simulink model "SHTL4_TestLevel_4_MODEL"  (R2017b)
settings: Solver=VariableStepAuto  StartTime=0.0  StopTime=80000000  RelTol=1e-3
libraries: instrumentlib x2, svdutilitieslib x1
settings Model: Creator=Bruger  LastModifiedBy=koch

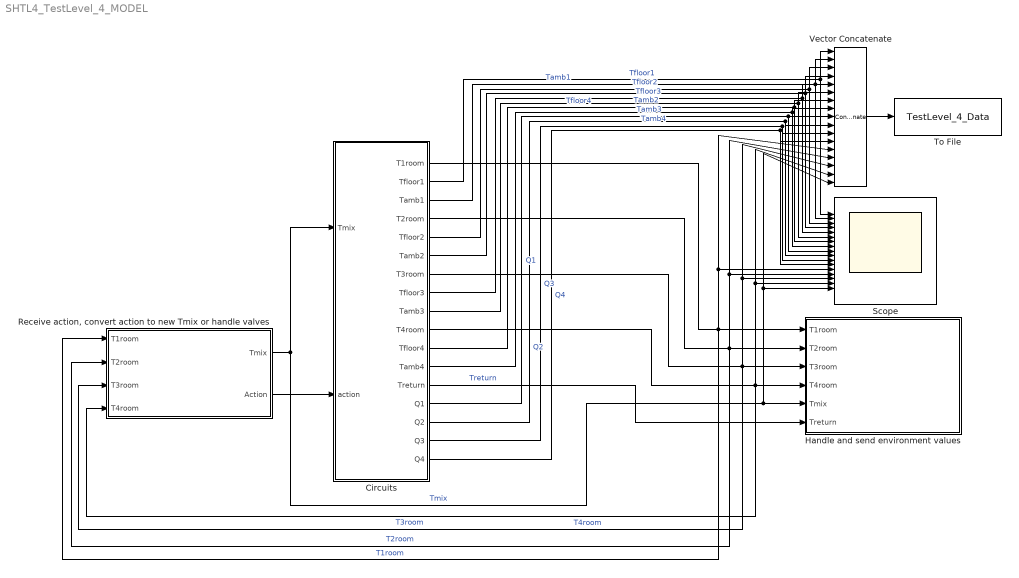
== system SHTL4_TestLevel_4_MODEL ==
  Circuits : Subsystem
  Handle and send environment values : Subsystem
  "Receive action, convert action to new Tmix or handle valves" : Subsystem
  Scope : Scope  NumInputPorts=17
  To File : ToFile  Filename=TestLevel_4_Data  SaveFormat=Timeseries
  Vector Concatenate : Concatenate  NumInputs=17
  wires:
  Vector Concatenate/1 -> To File/1
  "Receive action, convert action to new Tmix or handle valves"/1("Tmix ") -> Scope/17, Vector Concatenate/17, Handle and send environment values/5(Tmix), Circuits/1(Tmix)  "Tmix"
  "Receive action, convert action to new Tmix or handle valves"/2(Action) -> Circuits/2(action)
  Circuits/4(T2room) -> "Receive action, convert action to new Tmix or handle valves"/2(T2room), Scope/14, Vector Concatenate/14, Handle and send environment values/2(T2room)  "T2room"
  Circuits/7(T3room) -> "Receive action, convert action to new Tmix or handle valves"/3(T3room), Scope/15, Vector Concatenate/15, Handle and send environment values/3(T3room)  "T3room"
  Circuits/10(T4room) -> "Receive action, convert action to new Tmix or handle valves"/4(T4room), Scope/16, Vector Concatenate/16, Handle and send environment values/4(T4room)  "T4room"
  Circuits/1(T1room) -> "Receive action, convert action to new Tmix or handle valves"/1(T1room), Scope/13, Vector Concatenate/13, Handle and send environment values/1(T1room)  "T1room"
  Circuits/2(Tfloor1) -> Scope/1, Vector Concatenate/1  "Tfloor1"
  Circuits/3(Tamb1) -> Scope/2, Vector Concatenate/2  "Tamb1"
  Circuits/5(Tfloor2) -> Scope/3, Vector Concatenate/3  "Tfloor2"
  Circuits/6(Tamb2) -> Scope/4, Vector Concatenate/4  "Tamb2"
  Circuits/8(Tfloor3) -> Scope/5, Vector Concatenate/5  "Tfloor3"
  Circuits/9(Tamb3) -> Scope/6, Vector Concatenate/6  "Tamb3"
  Circuits/11(Tfloor4) -> Scope/7, Vector Concatenate/7  "Tfloor4"
  Circuits/12(Tamb4) -> Scope/8, Vector Concatenate/8  "Tamb4"
  Circuits/13(Treturn) -> Handle and send environment values/6(Treturn)  "Treturn"
  Circuits/14(Q1) -> Scope/9, Vector Concatenate/9  "Q1"
  Circuits/15(Q2) -> Scope/10, Vector Concatenate/10  "Q2"
  Circuits/16(Q3) -> Scope/11, Vector Concatenate/11  "Q3"
  Circuits/17(Q4) -> Scope/12, Vector Concatenate/12  "Q4"

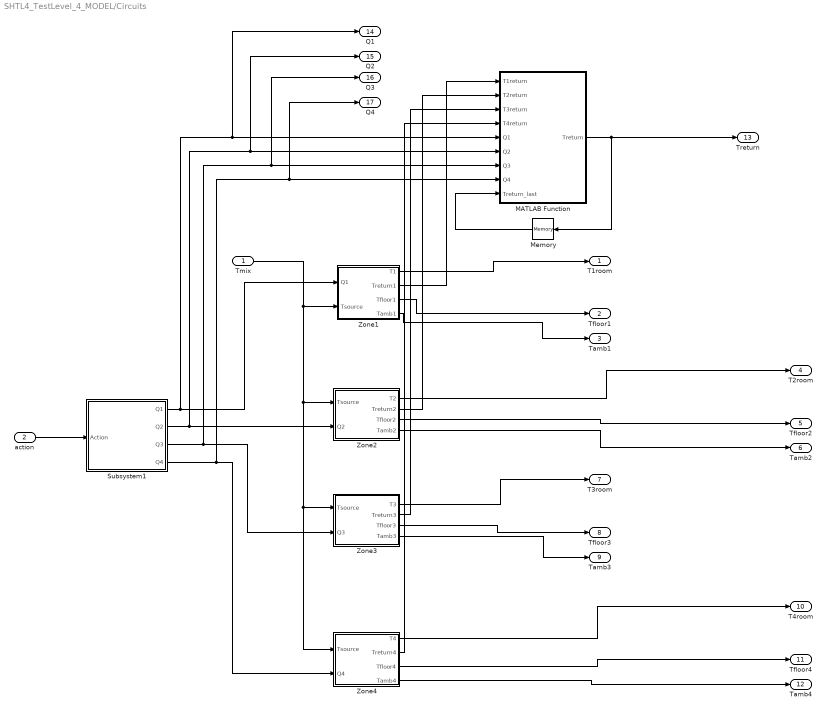
== system SHTL4_TestLevel_4_MODEL/Circuits ==
  Tmix : Inport
  action : Inport  Port=2
  MATLAB Function : MATLAB Function  TreatAsAtomicUnit=on
  Memory : Memory
  Subsystem1 : Subsystem
  Zone1 : Subsystem  Tag=Zone1  Description=Zone1
  Zone2 : Subsystem
  Zone3 : Subsystem
  Zone4 : Subsystem
  T1room : Outport
  Tfloor1 : Outport  Port=2
  Tamb1 : Outport  Port=3
  T2room : Outport  Port=4
  Tfloor2 : Outport  Port=5
  Tamb2 : Outport  Port=6
  T3room : Outport  Port=7
  Tfloor3 : Outport  Port=8
  Tamb3 : Outport  Port=9
  T4room : Outport  Port=10
  Tfloor4 : Outport  Port=11
  Tamb4 : Outport  Port=12
  Treturn : Outport  Port=13
  Q1 : Outport  Port=14
  Q2 : Outport  Port=15
  Q3 : Outport  Port=16
  Q4 : Outport  Port=17
  wires:
  Subsystem1/4("Q4 ") -> Q4/1, MATLAB Function/8(Q4), Zone4/2("Q4 ")
  action/1 -> Subsystem1/1("Action ")
  Tmix/1 -> Zone3/1(Tsource), Zone4/1(Tsource), Zone2/1(Tsource), Zone1/2(Tsource)
  Subsystem1/3(Q3) -> Q3/1, MATLAB Function/7(Q3), Zone3/2("Q3 ")
  Subsystem1/1("Q1 ") -> Q1/1, MATLAB Function/5(Q1), Zone1/1("Q1 ")
  Zone1/1(T1) -> T1room/1
  Zone1/2("Treturn1 ") -> MATLAB Function/1(T1return)
  Subsystem1/2(Q2) -> Q2/1, MATLAB Function/6(Q2), Zone2/2("Q2 ")
  Zone2/2("Treturn2 ") -> MATLAB Function/2(T2return)
  Zone3/2("Treturn3 ") -> MATLAB Function/3(T3return)
  Zone4/2(Treturn4) -> MATLAB Function/4(T4return)
  Zone1/3("Tfloor1 ") -> Tfloor1/1
  Zone1/4("Tamb1 ") -> Tamb1/1
  Zone2/1("T2 ") -> T2room/1
  Zone2/3("Tfloor2 ") -> Tfloor2/1
  Zone2/4("Tamb2 ") -> Tamb2/1
  Zone3/1(T3) -> T3room/1
  Zone3/3(Tfloor3) -> Tfloor3/1
  Zone3/4("Tamb3 ") -> Tamb3/1
  Zone4/1("T4 ") -> T4room/1
  Zone4/3("Tfloor4 ") -> Tfloor4/1
  Zone4/4("Tamb4 ") -> Tamb4/1
  MATLAB Function/1(Treturn) -> Treturn/1, Memory/1
  Memory/1 -> MATLAB Function/9(Treturn_last)

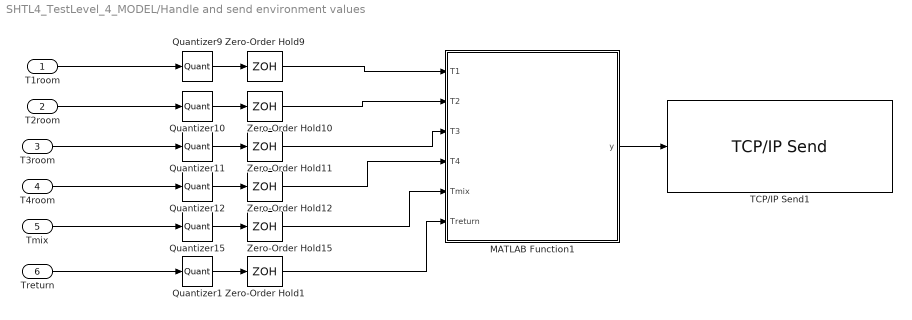
== system SHTL4_TestLevel_4_MODEL/Handle and send environment values ==
  T1room : Inport
  T2room : Inport  Port=2
  T3room : Inport  Port=3
  T4room : Inport  Port=4
  Tmix : Inport  Port=5
  Treturn : Inport  Port=6
  MATLAB Function1 : MATLAB Function  TreatAsAtomicUnit=on
  Quantizer{1,9..12,15} (6 alike) : Quantizer  QuantizationInterval=0.01
  TCP/IP Send1 : instrumentlib/TCP//IP Send  Host=localhost  Port=50001  EnableBlockingMode=on  Timeout=40  ByteOrder=LittleEndian
      settings: SourceProductName=Instrument Control Toolbox
  Zero-Order Hold{1,9..12,15} (6 alike) : ZeroOrderHold  SampleTime=-1
  wires:
  T4room/1 -> Quantizer12/1
  T1room/1 -> Quantizer9/1
  T3room/1 -> Quantizer11/1
  Tmix/1 -> Quantizer15/1
  T2room/1 -> Quantizer10/1
  Zero-Order Hold11/1 -> MATLAB Function1/3(T3)
  Quantizer11/1 -> Zero-Order Hold11/1
  Quantizer12/1 -> Zero-Order Hold12/1
  MATLAB Function1/1(y) -> TCP/IP Send1/1
  Zero-Order Hold10/1 -> MATLAB Function1/2(T2)
  Quantizer15/1 -> Zero-Order Hold15/1
  Zero-Order Hold12/1 -> MATLAB Function1/4(T4)
  Quantizer10/1 -> Zero-Order Hold10/1
  Zero-Order Hold9/1 -> MATLAB Function1/1(T1)
  Quantizer9/1 -> Zero-Order Hold9/1
  Zero-Order Hold15/1 -> MATLAB Function1/5(Tmix)
  Quantizer1/1 -> Zero-Order Hold1/1
  Treturn/1 -> Quantizer1/1
  Zero-Order Hold1/1 -> MATLAB Function1/6(Treturn)

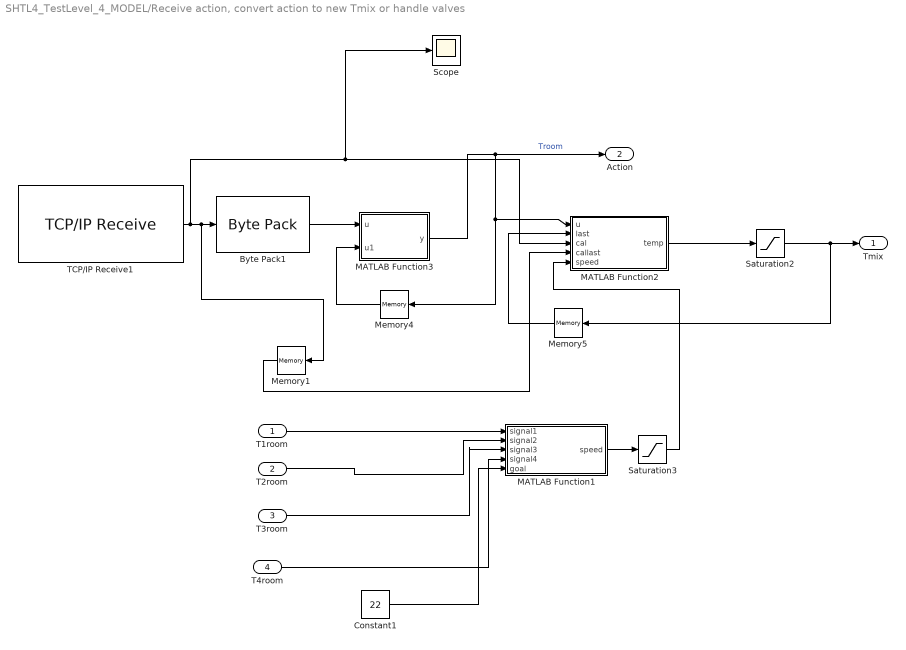
== system SHTL4_TestLevel_4_MODEL/Receive action, convert action to new Tmix or handle valves ==
  T1room : Inport
  T2room : Inport  Port=2
  T3room : Inport  Port=3
  T4room : Inport  Port=4
  Byte Pack1 : svdutilitieslib/Byte Pack  datatypes={'uint8'}  byteAlign=1  blockPlatform=arduinoert
      settings: SourceProductName=Simulink Support Package for Arduino Hardware  SourceProductBaseCode=ARDUINO
  Constant1 : Constant  Value=22
  MATLAB Function1 : MATLAB Function  TreatAsAtomicUnit=on
  MATLAB Function2 : MATLAB Function  TreatAsAtomicUnit=on
  MATLAB Function3 : MATLAB Function  TreatAsAtomicUnit=on
  Memory1 : Memory  InitialCondition=24
  Memory4 : Memory
  Memory5 : Memory  InitialCondition=24
  Saturation2 : Saturate  UpperLimit=45  LowerLimit=15
  Saturation3 : Saturate  UpperLimit=0.8  LowerLimit=0.005
  Scope : Scope
  TCP/IP Receive1 : instrumentlib/TCP//IP Receive  Host=localhost  Port=50000  DataSize=[1 1]  EnableBlockingMode=on  Timeout=40  SampleTime=200  DataType=uint8  ByteOrder=BigEndian
      settings: SourceProductName=Instrument Control Toolbox
  "Tmix " : Outport
  Action : Outport  Port=2
  wires:
  MATLAB Function1/1(speed) -> Saturation3/1
  Saturation3/1 -> MATLAB Function2/5(speed)
  MATLAB Function2/1(temp) -> Saturation2/1
  Byte Pack1/1 -> MATLAB Function3/1(u)
  MATLAB Function3/1(y) -> Action/1, Memory4/1, MATLAB Function2/1(u)  "Troom"
  TCP/IP Receive1/1 -> Scope/1, MATLAB Function2/3(cal), Memory1/1, Byte Pack1/1
  Memory4/1 -> MATLAB Function3/2(u1)
  Constant1/1 -> MATLAB Function1/5(goal)
  Memory5/1 -> MATLAB Function2/2(last)
  T1room/1 -> MATLAB Function1/1(signal1)
  T4room/1 -> MATLAB Function1/4(signal4)
  T3room/1 -> MATLAB Function1/3(signal3)
  T2room/1 -> MATLAB Function1/2(signal2)
  Saturation2/1 -> "Tmix "/1, Memory5/1
  Memory1/1 -> MATLAB Function2/4(callast)

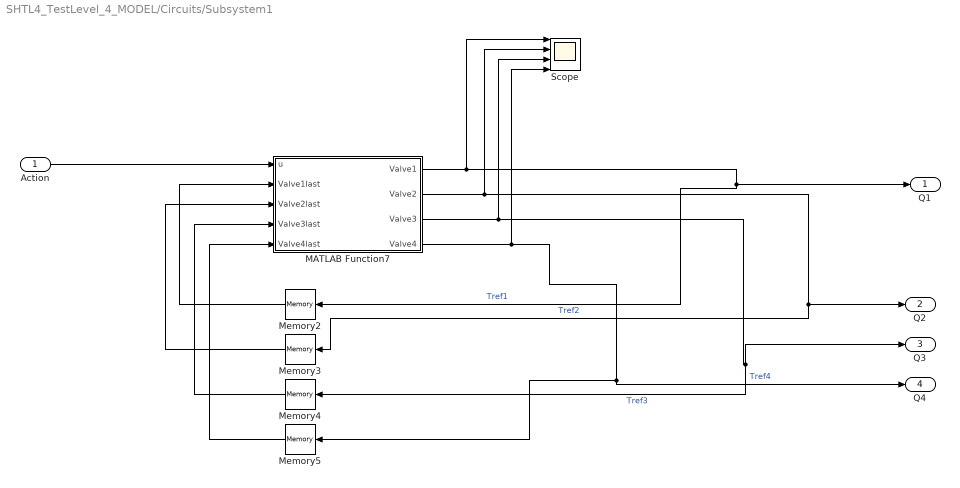
== system SHTL4_TestLevel_4_MODEL/Circuits/Subsystem1 ==
  "Action " : Inport
  MATLAB Function7 : MATLAB Function  TreatAsAtomicUnit=on
  Memory{2..5} (4 alike) : Memory  InitialCondition=0.000027777778
  Scope : Scope  NumInputPorts=4
  "Q1 " : Outport
  Q2 : Outport  Port=2
  Q3 : Outport  Port=3
  "Q4 " : Outport  Port=4
  wires:
  MATLAB Function7/4(Valve4) -> Scope/4, "Q4 "/1, Memory5/1  "Tref4"
  MATLAB Function7/3(Valve3) -> Scope/3, Q3/1, Memory4/1  "Tref3"
  MATLAB Function7/1(Valve1) -> Scope/1, Memory2/1, "Q1 "/1  "Tref1"
  MATLAB Function7/2(Valve2) -> Scope/2, Q2/1, Memory3/1  "Tref2"
  Memory5/1 -> MATLAB Function7/5(Valve4last)
  Memory2/1 -> MATLAB Function7/2(Valve1last)
  Memory4/1 -> MATLAB Function7/4(Valve3last)
  Memory3/1 -> MATLAB Function7/3(Valve2last)
  "Action "/1 -> MATLAB Function7/1(u)

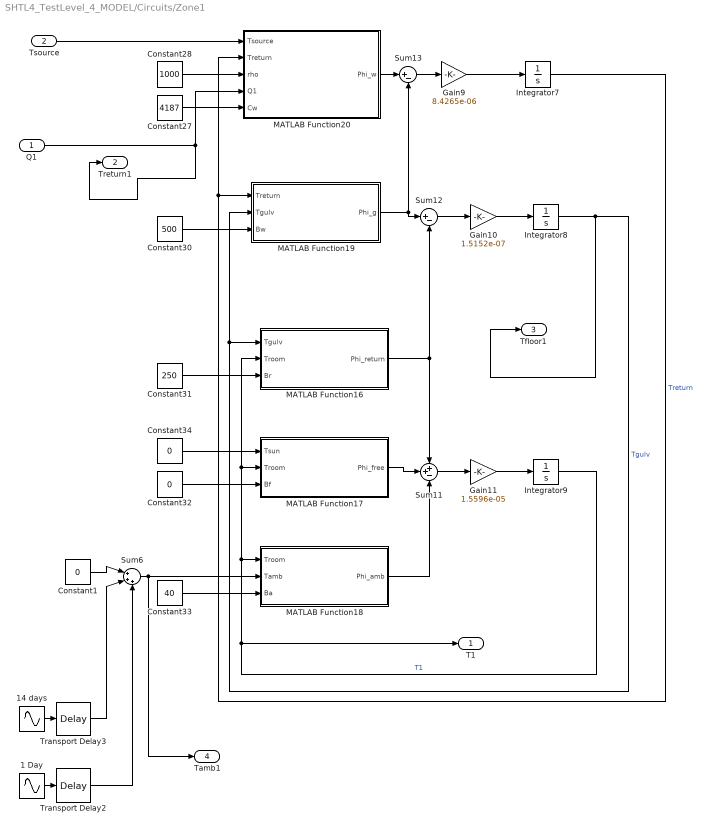
== system SHTL4_TestLevel_4_MODEL/Circuits/Zone1 ==
  "Q1 " : Inport
  Tsource : Inport  Port=2
  1 Day : Sin  Amplitude=4  Frequency=0.00007272205216643  SampleTime=0
  14 days : Sin  Amplitude=2  Frequency=0.00000519443  SampleTime=0
  Constant1 : Constant  Value=0
  Constant27 : Constant  Value=4187
  Constant28 : Constant  Value=1000
  Constant30 : Constant  Value=500
  Constant31 : Constant  Value=250
  Constant32 : Constant  Value=0
  Constant33 : Constant  Value=40
  Constant34 : Constant  Value=0
  Gain10 : Gain  Gain=1.5152e-07
  Gain11 : Gain  Gain=1.5596e-05
  Gain9 : Gain  Gain=8.4265e-06
  Integrator7 : Integrator  InitialCondition=15
  Integrator8 : Integrator  InitialCondition=15
  Integrator9 : Integrator  InitialCondition=15
  MATLAB Function16 : MATLAB Function  TreatAsAtomicUnit=on
  MATLAB Function17 : MATLAB Function  TreatAsAtomicUnit=on
  MATLAB Function18 : MATLAB Function  TreatAsAtomicUnit=on
  MATLAB Function19 : MATLAB Function  TreatAsAtomicUnit=on
  MATLAB Function20 : MATLAB Function  TreatAsAtomicUnit=on
  Sum11 : Sum  Inputs=++-
  Sum12 : Sum  Inputs=|+-
  Sum13 : Sum  Inputs=|+-
  Sum6 : Sum  Inputs=|+++
  Transport Delay2 : TransportDelay  DelayTime=15000000
  Transport Delay3 : TransportDelay  DelayTime=10000000
  T1 : Outport
  "Treturn1 " : Outport  Port=2
  "Tfloor1 " : Outport  Port=3
  "Tamb1 " : Outport  Port=4
  wires:
  Tsource/1 -> MATLAB Function20/1(Tsource)
  MATLAB Function20/1(Phi_w) -> Sum13/1
  Sum12/1 -> Gain10/1
  Constant31/1 -> MATLAB Function16/3(Br)
  Constant32/1 -> MATLAB Function17/3(Bf)
  Integrator7/1 -> MATLAB Function20/2(Treturn), MATLAB Function19/1(Treturn)  "Treturn"
  Gain11/1 -> Integrator9/1
  Constant33/1 -> MATLAB Function18/3(Ba)
  Gain9/1 -> Integrator7/1
  Constant34/1 -> MATLAB Function17/1(Tsun)
  Constant30/1 -> MATLAB Function19/3(Bw)
  Constant27/1 -> MATLAB Function20/5(Cw)
  Integrator9/1 -> T1/1, MATLAB Function16/2(Troom), MATLAB Function17/2(Troom), MATLAB Function18/1(Troom)  "T1"
  MATLAB Function18/1(Phi_amb) -> Sum11/3
  MATLAB Function19/1(Phi_g) -> Sum13/2, Sum12/1
  Sum11/1 -> Gain11/1
  Sum13/1 -> Gain9/1
  Integrator8/1 -> "Tfloor1 "/1, MATLAB Function16/1(Tgulv), MATLAB Function19/2(Tgulv)  "Tgulv"
  MATLAB Function16/1(Phi_return) -> Sum11/1, Sum12/2
  MATLAB Function17/1(Phi_free) -> Sum11/2
  Gain10/1 -> Integrator8/1
  Constant28/1 -> MATLAB Function20/3(rho)
  "Q1 "/1 -> "Treturn1 "/1, MATLAB Function20/4(Q1)
  Transport Delay2/1 -> Sum6/3
  14 days/1 -> Transport Delay3/1
  1 Day/1 -> Transport Delay2/1
  Constant1/1 -> Sum6/1
  Transport Delay3/1 -> Sum6/2
  Sum6/1 -> "Tamb1 "/1, MATLAB Function18/2(Tamb)

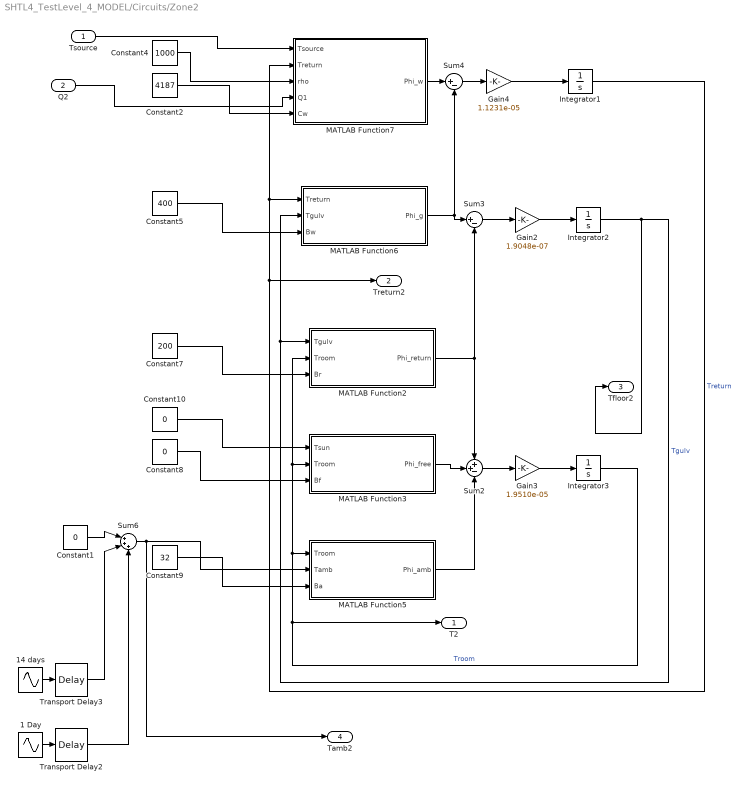
== system SHTL4_TestLevel_4_MODEL/Circuits/Zone2 ==
  Tsource : Inport
  "Q2 " : Inport  Port=2
  1 Day : Sin  Amplitude=4  Frequency=0.00007272205216643  SampleTime=0
  14 days : Sin  Amplitude=2  Frequency=0.00000519443  SampleTime=0
  Constant1 : Constant  Value=0
  Constant10 : Constant  Value=0
  Constant2 : Constant  Value=4187
  Constant4 : Constant  Value=1000
  Constant5 : Constant  Value=400
  Constant7 : Constant  Value=200
  Constant8 : Constant  Value=0
  Constant9 : Constant  Value=32
  Gain2 : Gain  Gain=1.9048e-07
  Gain3 : Gain  Gain=1.9510e-05
  Gain4 : Gain  Gain=1.1231e-05
  Integrator1 : Integrator  InitialCondition=15
  Integrator2 : Integrator  InitialCondition=15
  Integrator3 : Integrator  InitialCondition=15
  MATLAB Function2 : MATLAB Function  TreatAsAtomicUnit=on
  MATLAB Function3 : MATLAB Function  TreatAsAtomicUnit=on
  MATLAB Function5 : MATLAB Function  TreatAsAtomicUnit=on
  MATLAB Function6 : MATLAB Function  TreatAsAtomicUnit=on
  MATLAB Function7 : MATLAB Function  TreatAsAtomicUnit=on
  Sum2 : Sum  Inputs=++-
  Sum3 : Sum  Inputs=|+-
  Sum4 : Sum  Inputs=|+-
  Sum6 : Sum  Inputs=|+++
  Transport Delay2 : TransportDelay  DelayTime=15000000
  Transport Delay3 : TransportDelay  DelayTime=10000000
  "T2 " : Outport
  "Treturn2 " : Outport  Port=2
  "Tfloor2 " : Outport  Port=3
  "Tamb2 " : Outport  Port=4
  wires:
  Gain4/1 -> Integrator1/1
  Gain3/1 -> Integrator3/1
  MATLAB Function5/1(Phi_amb) -> Sum2/3
  Integrator2/1 -> "Tfloor2 "/1, MATLAB Function2/1(Tgulv), MATLAB Function6/2(Tgulv)  "Tgulv"
  Constant2/1 -> MATLAB Function7/5(Cw)
  MATLAB Function7/1(Phi_w) -> Sum4/1
  Sum4/1 -> Gain4/1
  Sum3/1 -> Gain2/1
  Integrator1/1 -> MATLAB Function7/2(Treturn), MATLAB Function6/1(Treturn), "Treturn2 "/1  "Treturn"
  Gain2/1 -> Integrator2/1
  MATLAB Function2/1(Phi_return) -> Sum2/1, Sum3/2
  Constant7/1 -> MATLAB Function2/3(Br)
  MATLAB Function6/1(Phi_g) -> Sum4/2, Sum3/1
  MATLAB Function3/1(Phi_free) -> Sum2/2
  Constant9/1 -> MATLAB Function5/3(Ba)
  Constant4/1 -> MATLAB Function7/3(rho)
  Integrator3/1 -> MATLAB Function2/2(Troom), MATLAB Function3/2(Troom), MATLAB Function5/1(Troom), "T2 "/1  "Troom"
  Sum2/1 -> Gain3/1
  Constant5/1 -> MATLAB Function6/3(Bw)
  "Q2 "/1 -> MATLAB Function7/4(Q1)
  Constant8/1 -> MATLAB Function3/3(Bf)
  Constant10/1 -> MATLAB Function3/1(Tsun)
  Tsource/1 -> MATLAB Function7/1(Tsource)
  Transport Delay2/1 -> Sum6/3
  14 days/1 -> Transport Delay3/1
  1 Day/1 -> Transport Delay2/1
  Constant1/1 -> Sum6/1
  Transport Delay3/1 -> Sum6/2
  Sum6/1 -> "Tamb2 "/1, MATLAB Function5/2(Tamb)

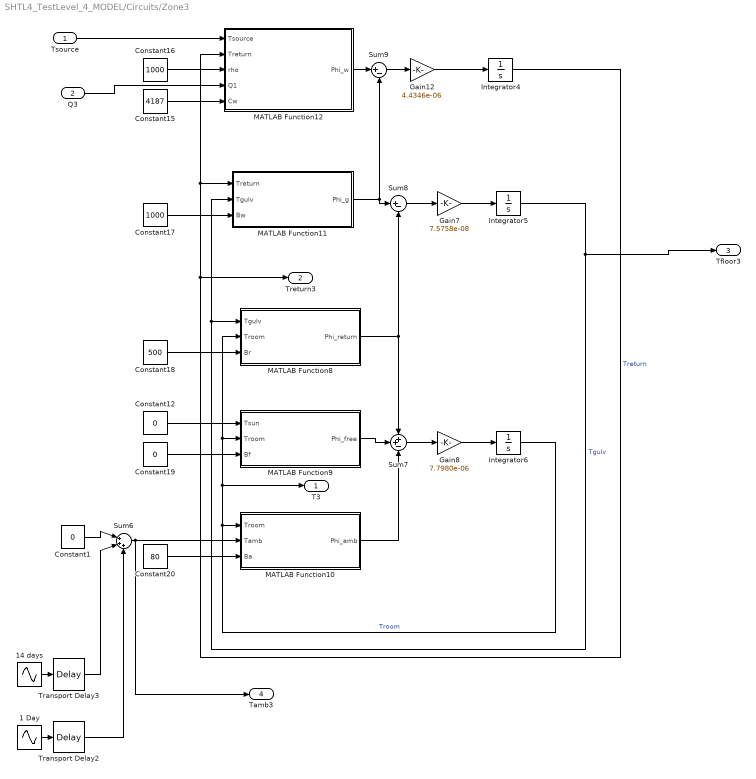
== system SHTL4_TestLevel_4_MODEL/Circuits/Zone3 ==
  Tsource : Inport
  "Q3 " : Inport  Port=2
  1 Day : Sin  Amplitude=4  Frequency=0.00007272205216643  SampleTime=0
  14 days : Sin  Amplitude=2  Frequency=0.00000519443  SampleTime=0
  Constant1 : Constant  Value=0
  Constant12 : Constant  Value=0
  Constant15 : Constant  Value=4187
  Constant16 : Constant  Value=1000
  Constant17 : Constant  Value=1000
  Constant18 : Constant  Value=500
  Constant19 : Constant  Value=0
  Constant20 : Constant  Value=80
  Gain12 : Gain  Gain=4.4346e-06
  Gain7 : Gain  Gain=7.5758e-08
  Gain8 : Gain  Gain=7.7980e-06
  Integrator4 : Integrator  InitialCondition=15
  Integrator5 : Integrator  InitialCondition=15
  Integrator6 : Integrator  InitialCondition=15
  MATLAB Function10 : MATLAB Function  TreatAsAtomicUnit=on
  MATLAB Function11 : MATLAB Function  TreatAsAtomicUnit=on
  MATLAB Function12 : MATLAB Function  TreatAsAtomicUnit=on
  MATLAB Function8 : MATLAB Function  TreatAsAtomicUnit=on
  MATLAB Function9 : MATLAB Function  TreatAsAtomicUnit=on
  Sum6 : Sum  Inputs=|+++
  Sum7 : Sum  Inputs=++-
  Sum8 : Sum  Inputs=|+-
  Sum9 : Sum  Inputs=|+-
  Transport Delay2 : TransportDelay  DelayTime=15000000
  Transport Delay3 : TransportDelay  DelayTime=10000000
  T3 : Outport
  "Treturn3 " : Outport  Port=2
  Tfloor3 : Outport  Port=3
  "Tamb3 " : Outport  Port=4
  wires:
  Constant17/1 -> MATLAB Function11/3(Bw)
  Integrator5/1 -> Tfloor3/1, MATLAB Function8/1(Tgulv), MATLAB Function11/2(Tgulv)  "Tgulv"
  MATLAB Function8/1(Phi_return) -> Sum7/1, Sum8/2
  Sum7/1 -> Gain8/1
  Gain7/1 -> Integrator5/1
  Constant16/1 -> MATLAB Function12/3(rho)
  MATLAB Function11/1(Phi_g) -> Sum9/2, Sum8/1
  Gain8/1 -> Integrator6/1
  Constant20/1 -> MATLAB Function10/3(Ba)
  MATLAB Function12/1(Phi_w) -> Sum9/1
  Integrator4/1 -> MATLAB Function12/2(Treturn), MATLAB Function11/1(Treturn), "Treturn3 "/1  "Treturn"
  Sum9/1 -> Gain12/1
  Constant15/1 -> MATLAB Function12/5(Cw)
  MATLAB Function10/1(Phi_amb) -> Sum7/3
  Constant19/1 -> MATLAB Function9/3(Bf)
  "Q3 "/1 -> MATLAB Function12/4(Q1)
  Sum8/1 -> Gain7/1
  Gain12/1 -> Integrator4/1
  Constant18/1 -> MATLAB Function8/3(Br)
  MATLAB Function9/1(Phi_free) -> Sum7/2
  Constant12/1 -> MATLAB Function9/1(Tsun)
  Integrator6/1 -> MATLAB Function10/1(Troom), MATLAB Function8/2(Troom), MATLAB Function9/2(Troom), T3/1  "Troom"
  Tsource/1 -> MATLAB Function12/1(Tsource)
  Transport Delay2/1 -> Sum6/3
  14 days/1 -> Transport Delay3/1
  1 Day/1 -> Transport Delay2/1
  Constant1/1 -> Sum6/1
  Transport Delay3/1 -> Sum6/2
  Sum6/1 -> "Tamb3 "/1, MATLAB Function10/2(Tamb)

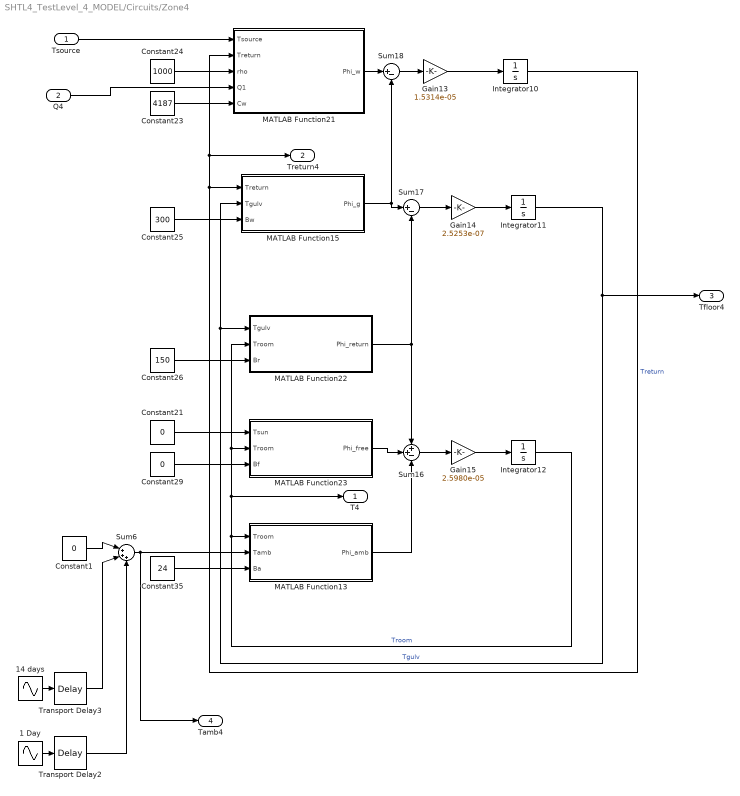
== system SHTL4_TestLevel_4_MODEL/Circuits/Zone4 ==
  Tsource : Inport
  "Q4 " : Inport  Port=2
  1 Day : Sin  Amplitude=4  Frequency=0.00007272205216643  SampleTime=0
  14 days : Sin  Amplitude=2  Frequency=0.00000519443  SampleTime=0
  Constant1 : Constant  Value=0
  Constant21 : Constant  Value=0
  Constant23 : Constant  Value=4187
  Constant24 : Constant  Value=1000
  Constant25 : Constant  Value=300
  Constant26 : Constant  Value=150
  Constant29 : Constant  Value=0
  Constant35 : Constant  Value=24
  Gain13 : Gain  Gain=1.5314e-05
  Gain14 : Gain  Gain=2.5253e-07
  Gain15 : Gain  Gain=2.5980e-05
  Integrator10 : Integrator  InitialCondition=15
  Integrator11 : Integrator  InitialCondition=15
  Integrator12 : Integrator  InitialCondition=15
  MATLAB Function13 : MATLAB Function  TreatAsAtomicUnit=on
  MATLAB Function15 : MATLAB Function  TreatAsAtomicUnit=on
  MATLAB Function21 : MATLAB Function  TreatAsAtomicUnit=on
  MATLAB Function22 : MATLAB Function  TreatAsAtomicUnit=on
  MATLAB Function23 : MATLAB Function  TreatAsAtomicUnit=on
  Sum16 : Sum  Inputs=++-
  Sum17 : Sum  Inputs=|+-
  Sum18 : Sum  Inputs=|+-
  Sum6 : Sum  Inputs=|+++
  Transport Delay2 : TransportDelay  DelayTime=15000000
  Transport Delay3 : TransportDelay  DelayTime=10000000
  "T4 " : Outport
  Treturn4 : Outport  Port=2
  "Tfloor4 " : Outport  Port=3
  "Tamb4 " : Outport  Port=4
  wires:
  Tsource/1 -> MATLAB Function21/1(Tsource)
  MATLAB Function22/1(Phi_return) -> Sum16/1, Sum17/2
  Sum18/1 -> Gain13/1
  Constant21/1 -> MATLAB Function23/1(Tsun)
  Sum6/1 -> "Tamb4 "/1, MATLAB Function13/2(Tamb)
  Integrator11/1 -> "Tfloor4 "/1, MATLAB Function22/1(Tgulv), MATLAB Function15/2(Tgulv)  "Tgulv"
  Constant25/1 -> MATLAB Function15/3(Bw)
  Constant29/1 -> MATLAB Function23/3(Bf)
  Integrator12/1 -> MATLAB Function13/1(Troom), MATLAB Function22/2(Troom), MATLAB Function23/2(Troom), "T4 "/1  "Troom"
  Gain14/1 -> Integrator11/1
  Integrator10/1 -> Treturn4/1, MATLAB Function21/2(Treturn), MATLAB Function15/1(Treturn)  "Treturn"
  Constant26/1 -> MATLAB Function22/3(Br)
  MATLAB Function13/1(Phi_amb) -> Sum16/3
  Sum17/1 -> Gain14/1
  MATLAB Function23/1(Phi_free) -> Sum16/2
  MATLAB Function21/1(Phi_w) -> Sum18/1
  MATLAB Function15/1(Phi_g) -> Sum18/2, Sum17/1
  "Q4 "/1 -> MATLAB Function21/4(Q1)
  Constant24/1 -> MATLAB Function21/3(rho)
  Constant23/1 -> MATLAB Function21/5(Cw)
  Constant35/1 -> MATLAB Function13/3(Ba)
  Sum16/1 -> Gain15/1
  Gain13/1 -> Integrator10/1
  Gain15/1 -> Integrator12/1
  Transport Delay2/1 -> Sum6/3
  14 days/1 -> Transport Delay3/1
  1 Day/1 -> Transport Delay2/1
  Constant1/1 -> Sum6/1
  Transport Delay3/1 -> Sum6/2

== matlab function SHTL4_TestLevel_4_MODEL/Circuits/MATLAB Function ==
  data: T1return input; Treturn output; T2return input; T3return input; T4return input; Q1 input; Q2 input; Q3 input; Q4 input; Treturn_last input
function Treturn = fcn(T1return, T2return, T3return, T4return, Q1, Q2, Q3, Q4, Treturn_last)

Treturn = (T1return * (Q1/(Q1+Q2+Q3+Q4))) + (T2return * (Q2/(Q1+Q2+Q3+Q4))) + (T3return * (Q3/(Q1+Q2+Q3+Q4))) + (T4return * (Q4/(Q1+Q2+Q3+Q4)));

if Q1 < 0.0000001 && Q2 < 0.0000001 && Q3 < 0.0000001 && Q4 < 0.0000001
    Treturn = Treturn_last;
end

== matlab function SHTL4_TestLevel_4_MODEL/Circuits/Zone1/MATLAB Function16 ==
  data: Tgulv input; Phi_return output; Troom input; Br input
function Phi_return = fcn(Tgulv,Troom,Br)

Phi_return = Br * ( Tgulv-Troom)

== matlab function SHTL4_TestLevel_4_MODEL/Circuits/Zone1/MATLAB Function17 ==
  data: Tsun input; Phi_free output; Troom input; Bf input
function Phi_free = fcn(Tsun,Troom,Bf)

Phi_free = Bf * ( Tsun-Troom)

== matlab function SHTL4_TestLevel_4_MODEL/Circuits/Zone1/MATLAB Function18 ==
  data: Troom input; Tamb input; Phi_amb output; Ba input
function Phi_amb = fcn(Troom,Tamb,Ba)

Phi_amb = Ba * ( Troom-Tamb)

== matlab function SHTL4_TestLevel_4_MODEL/Circuits/Zone1/MATLAB Function19 ==
  data: Treturn input; Tgulv input; Phi_g output; Bw input
function Phi_g= fcn(Treturn,Tgulv,Bw)

Phi_g = Bw * ( Treturn-Tgulv)

== matlab function SHTL4_TestLevel_4_MODEL/Circuits/Zone1/MATLAB Function20 ==
  data: Tsource input; Treturn input; Phi_w output; rho input; Q1 input; Cw input
function Phi_w= fcn(Tsource,Treturn,rho,Q1,Cw)

Phi_w = rho*Q1 *Cw* ( Tsource-Treturn)

== matlab function SHTL4_TestLevel_4_MODEL/Receive action, convert action to new Tmix or handle valves/MATLAB Function1 ==
  data: speed output; signal1 input; signal2 input; signal3 input; signal4 input; goal input
function speed = fcn(signal1,signal2,signal3,signal4, goal)

delta1 =abs(goal - signal1)
delta2 =abs(goal - signal2)
delta3 =abs(goal - signal3)
delta4 =abs(goal - signal4)

Delta = [delta1;delta2;delta3;delta4]

if goal > 0 && signal1 > 0
speed = min(Delta)*0.3
else 
    speed = 0.1
end

if speed < 0.03
    speed =0.03
end

== matlab function SHTL4_TestLevel_4_MODEL/Receive action, convert action to new Tmix or handle valves/MATLAB Function2 ==
  data: u input; temp output; last input; cal input; callast input; speed input
function temp= fcn(u,last,cal,callast,speed)



    if cal > callast 
         k=1
    else
        k=0
    end


if u < 2 && k>0
temp = last
k=0
elseif 1 < u && u < 3 && k>0
    temp=last - speed
    k=0
elseif 2 < u && k>0 && u < 4
    temp = last+speed
    k=0
elseif u > 20
    temp = u;
else
    temp=last
    k=0
end

== matlab function SHTL4_TestLevel_4_MODEL/Receive action, convert action to new Tmix or handle valves/MATLAB Function3 ==
  data: u input; y output; u1 input
function y  = fcn(u,u1)

u = double(u);
% zero is not a option so
if u > 0
    y = u;
else
    y = u1;
end

== matlab function SHTL4_TestLevel_4_MODEL/Circuits/Zone2/MATLAB Function2 ==
  data: Tgulv input; Phi_return output; Troom input; Br input
function Phi_return = fcn(Tgulv,Troom,Br)

Phi_return = Br * ( Tgulv-Troom)

== matlab function SHTL4_TestLevel_4_MODEL/Circuits/Subsystem1/MATLAB Function7 ==
  data: u input; Valve1 output; Valve2 output; Valve1last input; Valve2last input; Valve3last input; Valve4last input; Valve3 output; Valve4 output
function [Valve1,Valve2,Valve3,Valve4]= fcn(u,Valve1last,Valve2last,Valve3last,Valve4last)
if u < 4
    Valve1 = Valve1last
    Valve2 = Valve2last
    Valve3 = Valve3last
    Valve4 = Valve4last
elseif u > 3 && 5 > u % u = 4
    Valve1 = (2.77777778 * 10^-5)*2 
    Valve2 = (2.77777778 * 10^-5)*2 
    Valve3 = (2.77777778 * 10^-5)*2 
    Valve4 = (2.77777778 * 10^-5)*2 
elseif u > 4 && 6 > u % u = 5
    Valve1 = (2.77777778 * 10^-5)*2 
    Valve2 = 0
    Valve3 = 0
    Valve4 = 0
elseif u > 5 && 7 > u % u = 6
    Valve1 = 0
    Valve2 = (2.77777778 * 10^-5)*2
    Valve3 = 0
    Valve4 = 0
elseif u > 6 && 8 > u % u = 7
    Valve1 = 0
    Valve2 = 0
    Valve3 = (2.77777778 * 10^-5)*2
    Valve4 = 0
elseif u > 7 && 9 > u % u = 8
    Valve1 = 0
    Valve2 = 0
    Valve3 = 0
    Valve4 = (2.77777778 * 10^-5)*2
elseif u > 8 && 10 > u % u = 9
    Valve1 = (2.77777778 * 10^-5)*2
    Valve2 = (2.77777778 * 10^-5)*2
    Valve3 = 0
    Valve4 = 0
elseif u > 9 && 11 > u % u = 10
    Valve1 = 0
    Valve2 = (2.77777778 * 10^-5)*2
    Valve3 = (2.77777778 * 10^-5)*2
    Valve4 = 0
elseif u > 10 && 12 > u % u = 11
    Valve1 = 0
    Valve2 = 0
    Valve3 = (2.77777778 * 10^-5)*2
    Valve4 = (2.77777778 * 10^-5)*2
elseif u > 11 && 13 > u % u = 12
    Valve1 = (2.77777778 * 10^-5)*2
    Valve2 = 0
    Valve3 = 0
    Valve4 = (2.77777778 * 10^-5)*2
elseif u > 12 && 14 > u % u = 13
    Valve1 = (2.77777778 * 10^-5)*2
    Valve2 = 0
    Valve3 = (2.77777778 * 10^-5)*2
    Valve4 = 0
elseif u > 13 && 15 > u % u = 14
    Valve1 = 0
    Valve2 = (2.77777778 * 10^-5)*2
    Valve3 = 0
    Valve4 = (2.77777778 * 10^-5)*2
elseif u > 14 && 16 > u % u = 15
    Valve1 = (2.77777778 * 10^-5)*2
    Valve2 = (2.77777778 * 10^-5)*2
    Valve3 = (2.77777778 * 10^-5)*2
    Valve4 = 0
elseif u > 15 && 17 > u % u = 16
    Valve1 = (2.77777778 * 10^-5)*2
    Valve2 = (2.77777778 * 10^-5)*2
    Valve3 = 0
    Valve4 = (2.77777778 * 10^-5)*2
elseif u > 16 && 18 > u % u = 17
    Valve1 = (2.77777778 * 10^-5)*2
    Valve2 = 0
    Valve3 = (2.77777778 * 10^-5)*2
    Valve4 = (2.77777778 * 10^-5)*2
elseif u > 17 && 19 > u % u = 18
    Valve1 = 0
    Valve2 = (2.77777778 * 10^-5)*2
    Valve3 = (2.77777778 * 10^-5)*2
    Valve4 = (2.77777778 * 10^-5)*2
elseif u > 18 && 20 > u % u = 19
    Valve1 = 0
    Valve2 = 0
    Valve3 = 0
    Valve4 = 0
else 
    Valve1 = Valve1last
    Valve2 = Valve2last
    Valve3 = Valve3last
    Valve4 = Valve4last
end

== matlab function SHTL4_TestLevel_4_MODEL/Handle and send environment values/MATLAB Function1 ==
  data: T1 input; y output; T2 input; T3 input; T4 input; Tmix input; Treturn input
function y = fcn(T1,T2,T3,T4,Tmix, Treturn)

y = [T1, T2, T3, T4, Tmix, Treturn];

== matlab function SHTL4_TestLevel_4_MODEL/Circuits/Zone2/MATLAB Function3 ==
  data: Tsun input; Phi_free output; Troom input; Bf input
function Phi_free = fcn(Tsun,Troom,Bf)

Phi_free = Bf * ( Tsun-Troom)

== matlab function SHTL4_TestLevel_4_MODEL/Circuits/Zone2/MATLAB Function5 ==
  data: Troom input; Tamb input; Phi_amb output; Ba input
function Phi_amb = fcn(Troom,Tamb,Ba)

Phi_amb = Ba * ( Troom-Tamb)

== matlab function SHTL4_TestLevel_4_MODEL/Circuits/Zone2/MATLAB Function6 ==
  data: Treturn input; Tgulv input; Phi_g output; Bw input
function Phi_g= fcn(Treturn,Tgulv,Bw)

Phi_g = Bw * ( Treturn-Tgulv)

== matlab function SHTL4_TestLevel_4_MODEL/Circuits/Zone2/MATLAB Function7 ==
  data: Tsource input; Treturn input; Phi_w output; rho input; Q1 input; Cw input
function Phi_w= fcn(Tsource,Treturn,rho,Q1,Cw)

Phi_w = rho*Q1*0.8 *Cw* ( Tsource-Treturn)

== matlab function SHTL4_TestLevel_4_MODEL/Circuits/Zone3/MATLAB Function10 ==
  data: Troom input; Tamb input; Phi_amb output; Ba input
function Phi_amb = fcn(Troom,Tamb,Ba)

Phi_amb = Ba * ( Troom-Tamb)

== matlab function SHTL4_TestLevel_4_MODEL/Circuits/Zone3/MATLAB Function11 ==
  data: Treturn input; Tgulv input; Phi_g output; Bw input
function Phi_g= fcn(Treturn,Tgulv,Bw)

Phi_g = Bw * ( Treturn-Tgulv)

== matlab function SHTL4_TestLevel_4_MODEL/Circuits/Zone3/MATLAB Function12 ==
  data: Tsource input; Treturn input; Phi_w output; rho input; Q1 input; Cw input
function Phi_w= fcn(Tsource,Treturn,rho,Q1,Cw)

Phi_w = rho*Q1*2.5 *Cw* ( Tsource-Treturn)

== matlab function SHTL4_TestLevel_4_MODEL/Circuits/Zone3/MATLAB Function8 ==
  data: Tgulv input; Phi_return output; Troom input; Br input
function Phi_return = fcn(Tgulv,Troom,Br)

Phi_return = Br * ( Tgulv-Troom)

== matlab function SHTL4_TestLevel_4_MODEL/Circuits/Zone3/MATLAB Function9 ==
  data: Tsun input; Phi_free output; Troom input; Bf input
function Phi_free = fcn(Tsun,Troom,Bf)

Phi_free = Bf * ( Tsun-Troom)

== matlab function SHTL4_TestLevel_4_MODEL/Circuits/Zone4/MATLAB Function13 ==
  data: Troom input; Tamb input; Phi_amb output; Ba input
function Phi_amb = fcn(Troom,Tamb,Ba)

Phi_amb = Ba * ( Troom-Tamb)

== matlab function SHTL4_TestLevel_4_MODEL/Circuits/Zone4/MATLAB Function15 ==
  data: Treturn input; Tgulv input; Phi_g output; Bw input
function Phi_g= fcn(Treturn,Tgulv,Bw)

Phi_g = Bw * ( Treturn-Tgulv)

== matlab function SHTL4_TestLevel_4_MODEL/Circuits/Zone4/MATLAB Function21 ==
  data: Tsource input; Treturn input; Phi_w output; rho input; Q1 input; Cw input
function Phi_w= fcn(Tsource,Treturn,rho,Q1,Cw)

Phi_w = rho*Q1*0.6 *Cw* ( Tsource-Treturn)

== matlab function SHTL4_TestLevel_4_MODEL/Circuits/Zone4/MATLAB Function22 ==
  data: Tgulv input; Phi_return output; Troom input; Br input
function Phi_return = fcn(Tgulv,Troom,Br)

Phi_return = Br * ( Tgulv-Troom)

== matlab function SHTL4_TestLevel_4_MODEL/Circuits/Zone4/MATLAB Function23 ==
  data: Tsun input; Phi_free output; Troom input; Bf input
function Phi_free = fcn(Tsun,Troom,Bf)

Phi_free = Bf * ( Tsun-Troom)
